simulink model "Linear_Trajectory_Tracking_Simulink"  (R2024b)
settings: Solver=VariableStepAuto  StartTime=0.0  StopTime=10.0  RelTol=1e-3
values from neighbouring files (symbols this model uses):
  a = 3    [constants.m]
  xi = 0.6    [constants.m]
settings Model: Creator=emica  LastModifiedBy=emica

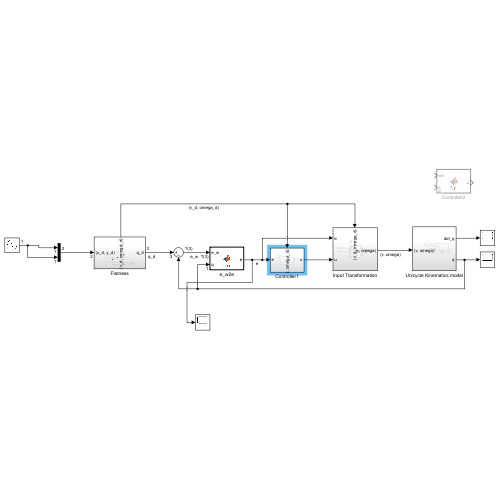
[thumbnail: Simulink's stored preview of the top-level diagram]
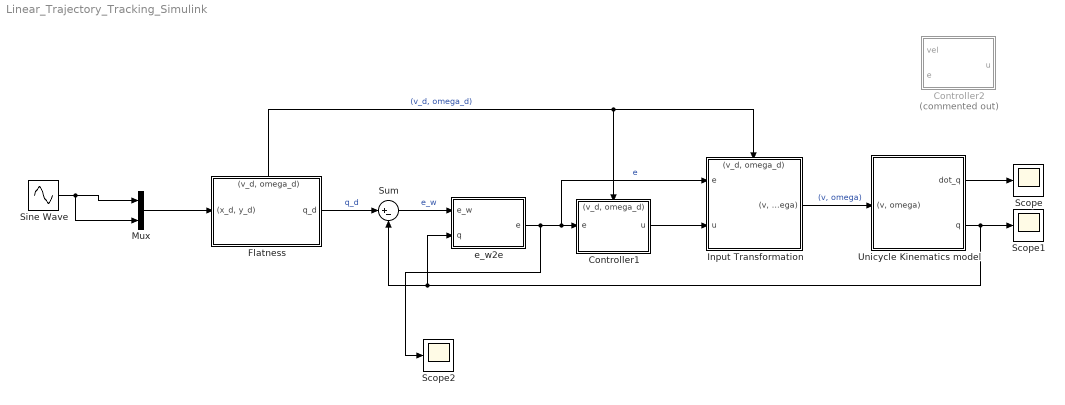
== system Linear_Trajectory_Tracking_Simulink ==
  Controller1 : Subsystem
      settings: PortSchema="{\"entries\":[{\"content\":{\"sides\":[{\"content\":{\"connectorIds\":[\"In1\"]},\"type\":\"ConnectorPlacement.EquallySpacedRectSide\",\"uuid\":\"663a145a-b0a1-462d-957e-da25aa8d70ec\"},{\"content\":{\"connectorIds\":[\"Out1\"],\"side\":\"RIGHT\"},\"type\":\"ConnectorPlacement.EquallySpacedRectSide\",\"uuid\":\"3d00da72-66aa-4dae-9c0c-49820669bfbe\"},{\"content\":{\"connectorIds\":[\"In2\"],\"side\":\"TOP\"},\"type\":\"ConnectorPlacement.EquallySpacedRectSide\",\"uuid\":\"8e215669-d1a4-45b0-90e4-6e6fca69e90d\"}]},\"type\":\"ConnectorPlacement.EquallySpacedConnector\",\"uuid\":\"7b416759-2a96-476f-93d6-d6b19fa598e9\"}],\"packageUris\":[\"http://schema.mathworks.com/mf0/Connector/R2020b\"],\"version\":\"1.0\"}"
  Controller2 : MATLAB Function  Commented=on  TreatAsAtomicUnit=on
  Flatness : Subsystem
      settings: PortSchema="{\"entries\":[{\"content\":{\"sides\":[{\"content\":{\"connectorIds\":[\"In1\"]},\"type\":\"ConnectorPlacement.EquallySpacedRectSide\",\"uuid\":\"bc490c8e-5666-439b-9939-62bd84628b1f\"},{\"content\":{\"connectorIds\":[\"Out1\"],\"side\":\"RIGHT\"},\"type\":\"ConnectorPlacement.EquallySpacedRectSide\",\"uuid\":\"03a20fcc-2a82-4af2-a970-ff3426fda7d9\"},{\"content\":{\"connectorIds\":[\"Out2\"],\"side\":\"TOP\"},\"type\":\"ConnectorPlacement.EquallySpacedRectSide\",\"uuid\":\"09224fef-e39c-4959-bd2b-02867a510190\"}]},\"type\":\"ConnectorPlacement.EquallySpacedConnector\",\"uuid\":\"ad9510e9-14f7-413e-ab85-da35fb962608\"}],\"packageUris\":[\"http://schema.mathworks.com/mf0/Connector/R2020b\"],\"version\":\"1.0\"}"
  Input Transformation : Subsystem
      settings: PortSchema="{\"entries\":[{\"content\":{\"sides\":[{\"content\":{\"connectorIds\":[\"In1\",\"In2\"]},\"type\":\"ConnectorPlacement.EquallySpacedRectSide\",\"uuid\":\"4cbebdc1-8913-4bb0-9524-d854c819f784\"},{\"content\":{\"connectorIds\":[\"Out1\"],\"side\":\"RIGHT\"},\"type\":\"ConnectorPlacement.EquallySpacedRectSide\",\"uuid\":\"178a2b4a-0c33-47f3-8be3-bd76dfc47961\"},{\"content\":{\"connectorIds\":[\"In3\"],\"side\":\"TOP\"},\"type\":\"ConnectorPlacement.EquallySpacedRectSide\",\"uuid\":\"3e37ae07-0719-4d1d-ac53-f79374967c51\"}]},\"type\":\"ConnectorPlacement.EquallySpacedConnector\",\"uuid\":\"35111781-18f4-42cf-8750-882b65aa13c0\"}],\"packageUris\":[\"http://schema.mathworks.com/mf0/Connector/R2020b\"],\"version\":\"1.0\"}"
  Mux : Mux  Inputs=2
  Scope : Scope
  Scope1 : Scope
  Scope2 : Scope
  Sine Wave : Sin  SampleTime=0
  Sum : Sum  Inputs=|+-
  Unicycle Kinematics model : Subsystem
  e_w2e : MATLAB Function  TreatAsAtomicUnit=on
  wires:
  Mux/1 -> Flatness/1("(x_d, y_d)")
  Flatness/2("(v_d, omega_d)") -> Input Transformation/3("(v_d, omega_d)"), Controller1/2("(v_d, omega_d)")  "(v_d, omega_d)"
  Sum/1 -> e_w2e/1(e_w)  "e_w"
  Unicycle Kinematics model/2(q) -> e_w2e/2(q), Sum/2, Scope1/1
  e_w2e/1(e) -> Scope2/1, Controller1/1(e), Input Transformation/1(e)  "e"
  Controller1/1(u) -> Input Transformation/2(u)
  Input Transformation/1("(v, omega)") -> Unicycle Kinematics model/1("(v, omega)")  "(v, omega)"
  Unicycle Kinematics model/1(dot_q) -> Scope/1
  Sine Wave/1 -> Mux/2, Mux/1
  Flatness/1(q_d) -> Sum/1  "q_d"

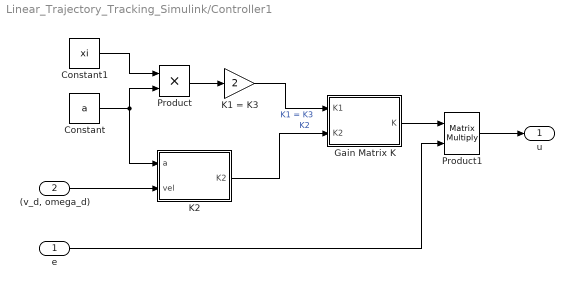
== system Linear_Trajectory_Tracking_Simulink/Controller1 ==
  e : Inport
  "(v_d, omega_d)" : Inport  Port=2
  Constant : Constant  Value=a
  Constant1 : Constant  Value=xi
  Gain Matrix K : MATLAB Function  TreatAsAtomicUnit=on
  K1 = K3 : Gain  Gain=2
  K2 : MATLAB Function  TreatAsAtomicUnit=on
  Product : Product
  Product1 : Product  Multiplication=Matrix(*)
  u : Outport
  wires:
  e/1 -> Product1/2
  Gain Matrix K/1(K) -> Product1/1
  Product1/1 -> u/1
  K2/1(K2) -> Gain Matrix K/2(K2)  "K2"
  K1 = K3/1 -> Gain Matrix K/1(K1)  "K1 = K3"
  Constant/1 -> K2/1(a), Product/2
  Constant1/1 -> Product/1
  "(v_d, omega_d)"/1 -> K2/2(vel)
  Product/1 -> K1 = K3/1

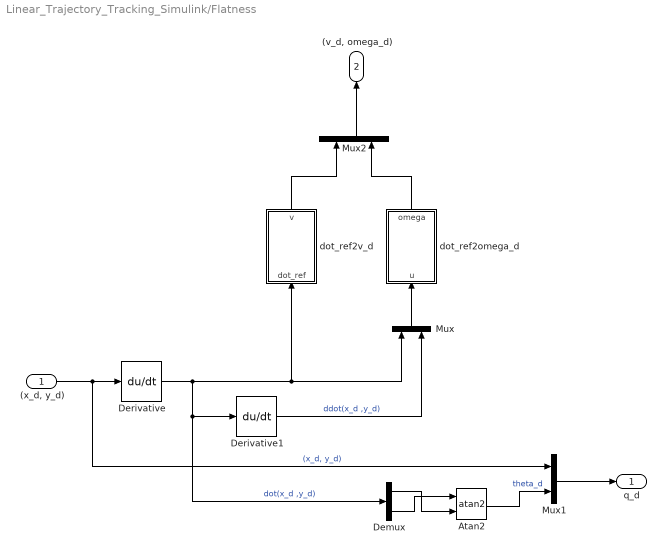
== system Linear_Trajectory_Tracking_Simulink/Flatness ==
  "(x_d, y_d)" : Inport
  Atan2 : Trigonometry  Operator=atan2
  Demux : Demux  Outputs=2
  Derivative : Derivative
  Derivative1 : Derivative
  Mux : Mux  Inputs=2
  Mux1 : Mux  Inputs=2
  Mux2 : Mux  Inputs=2
  dot_ref2omega_d : MATLAB Function  TreatAsAtomicUnit=on
  dot_ref2v_d : MATLAB Function  TreatAsAtomicUnit=on
  q_d : Outport
  "(v_d, omega_d)" : Outport  Port=2
  wires:
  Atan2/1 -> Mux1/2  "theta_d"
  "(x_d, y_d)"/1 -> Mux1/1, Derivative/1  "(x_d, y_d)"
  Mux/1 -> dot_ref2omega_d/1(u)
  Derivative/1 -> Mux/1, dot_ref2v_d/1(dot_ref), Demux/1, Derivative1/1  "dot(x_d ,y_d)"
  Demux/1 -> Atan2/2
  Derivative1/1 -> Mux/2  "ddot(x_d ,y_d)"
  Demux/2 -> Atan2/1
  Mux1/1 -> q_d/1
  Mux2/1 -> "(v_d, omega_d)"/1
  dot_ref2omega_d/1(omega) -> Mux2/2
  dot_ref2v_d/1(v) -> Mux2/1

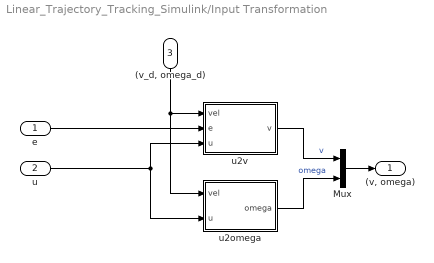
== system Linear_Trajectory_Tracking_Simulink/Input Transformation ==
  e : Inport
  u : Inport  Port=2
  "(v_d, omega_d)" : Inport  Port=3
  Mux : Mux  Inputs=2
  u2omega : MATLAB Function  TreatAsAtomicUnit=on
  u2v : MATLAB Function  TreatAsAtomicUnit=on
  "(v, omega)" : Outport
  wires:
  e/1 -> u2v/2(e)
  Mux/1 -> "(v, omega)"/1
  u2omega/1(omega) -> Mux/2  "omega"
  u2v/1(v) -> Mux/1  "v"
  u/1 -> u2omega/2(u), u2v/3(u)
  "(v_d, omega_d)"/1 -> u2v/1(vel), u2omega/1(vel)

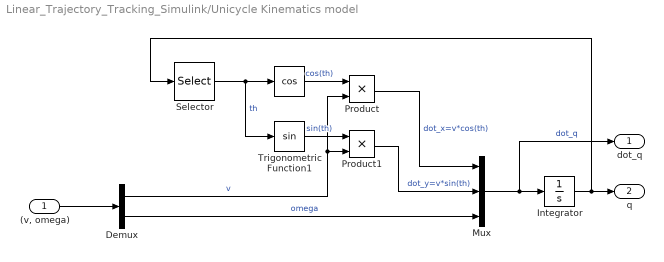
== system Linear_Trajectory_Tracking_Simulink/Unicycle Kinematics model ==
  "(v, omega)" : Inport
  " " : Trigonometry  Operator=cos
  Demux : Demux  Outputs=2
  Integrator : Integrator  InitialCondition=1e-10
  Mux : Mux  Inputs=3
  Product : Product
  Product1 : Product
  Selector : Selector  InputPortWidth=3  IndexOptions=Index vector (dialog)  Indices=[3]  OutputSizes=1
  Trigonometric Function1 : Trigonometry
  dot_q : Outport
  q : Outport  Port=2
  wires:
  Integrator/1 -> Selector/1, q/1
  "(v, omega)"/1 -> Demux/1
  Mux/1 -> dot_q/1, Integrator/1  "dot_q"
  Demux/2 -> Mux/3  "omega"
  Selector/1 -> Trigonometric Function1/1, " "/1  "th"
  " "/1 -> Product/1  "cos(th)"
  Trigonometric Function1/1 -> Product1/1  "sin(th)"
  Demux/1 -> Product1/2, Product/2  "v"
  Product1/1 -> Mux/2  "dot_y=v*sin(th)"
  Product/1 -> Mux/1  "dot_x=v*cos(th)"

== matlab function Linear_Trajectory_Tracking_Simulink/Flatness/dot_ref2v_d ==
  data: dot_ref input; v output
function v = fcn(dot_ref)
    dot_x = dot_ref(1);
    dot_y = dot_ref(2);

    v = sqrt(dot_x^2 + dot_y^2);

== matlab function Linear_Trajectory_Tracking_Simulink/e_w2e ==
  data: e_w input; e output; q input
function e = fcn(e_w, q)
    theta = q(3);

    R = [cos(theta) sin(theta) 0; 
        -sin(theta) cos(theta) 0;
             0          0      1];

    e = R*e_w;

== matlab function Linear_Trajectory_Tracking_Simulink/Controller1/Gain Matrix K ==
  data: K1 input; K output; K2 input
function K = fcn(K1, K2)
K3 = K1;

K = [-K1  0   0;
      0  -K2 -K3];

== matlab function Linear_Trajectory_Tracking_Simulink/Controller1/K2 ==
  data: a input; vel input; K2 output
function K2 = fcn(a, vel)
v_d = vel(1);
omega_d = vel(2);

K2 = (a^2-omega_d^2)/(v_d);

== matlab function Linear_Trajectory_Tracking_Simulink/Controller2 ==
  data: vel input; u output; e input
function u = fcn(vel, e)

d = 1/sqrt(2);
a = 10;
v_d = vel(1);
omega_d = vel(2);

k1 = 2*d*a;
if abs(v_d) < 1e-4
    if v_d >= 0
        v_d = 1e-4;
    else
        v_d = -1e-4;
        
    end
end
k2 = (a^2 - omega_d^2)/v_d;
k3 = k1;
k = [-k1,0,0; 0, -k2, -k3];

u = k*e;

== matlab function Linear_Trajectory_Tracking_Simulink/Input Transformation/u2omega ==
  data: vel input; u input; omega output
function omega = fcn(vel,u)
    omega_d = vel(2);

    omega = omega_d-u(2);

== matlab function Linear_Trajectory_Tracking_Simulink/Input Transformation/u2v ==
  data: vel input; e input; u input; v output
function v = fcn(vel, e, u)
 v_d = vel(1);

 v = v_d*cos(e(3))-u(1);

== matlab function Linear_Trajectory_Tracking_Simulink/Flatness/dot_ref2omega_d ==
  data: u input; omega output
function omega = fcn(u)
    dot_x = u(1);
    dot_y = u(2);
    ddot_x = u(3);
    ddot_y = u(4);

    omega = (dot_x*ddot_y - dot_y*ddot_x) / (dot_x^2 + dot_y^2);
